simulink model "qubeLQGR_discrete_distrej"  (R2024b)
settings: Solver=ode1  StartTime=0.0  StopTime=120  RelTol=1e-3  EnableMultiTasking=on
values from neighbouring files (symbols this model uses):
  epsilon = 0.00242    [MPC_controller.m]    (also in MPC_controller_withint_testing.m)
  h = log(abs(sec(theta)+tan(theta))-C1*alpha)    [Design_of_nonlinear_controller.m]    (also in MPC_controller.m = 0.01; MPC_controller_withint_testing.m = 0.01)
undefined symbols (not defined in the file or in its folder): Discrete, Humusoft, MF634, Time
libraries: sldrtlib x2, simulink x2, ctrlSharedLib x1
settings Model: Creator=rbabuska  LastModifiedBy=Wesley
settings SolverCC: AlgebraicLoopSolver=TrustRegion
settings DataIOCC: LimitDataPoints=on  SaveFormat=Array  SignalLoggingSaveFormat=ModelDataLogs  ReturnWorkspaceOutputs=off
settings OptimizationCC: ExpressionDepthLimit=2147483647  LifeSpan=inf
settings DebuggingCC: UnderspecifiedInitializationDetection=Classic  MergeDetectMultiDrivingBlocksExec=none  FcnCallInpInsideContextMsg=warning  UnconnectedInputMsg=warning  UnconnectedOutputMsg=warning  UnconnectedLineMsg=warning  StateNameClashWarn=warning  SFUnexpectedBacktrackingDiag=warning  SFNoUnconditionalDefaultTransitionDiag=warning  SFExecutionAtInitializationDiag=none  ArithmeticOperatorsInVariantConditions=warning
settings HardwareCC: ProdBitPerPointer=32  ProdBitPerSizeT=32  ProdBitPerPtrDiffT=32  ProdLargestAtomicFloat=None  ProdIntDivRoundTo=Undefined  ProdEndianess=Unspecified  ProdWordSize=32  ProdHWDeviceType=32-bit Generic
settings ModelReferenceCC: EnableRefExpFcnMdlSchedulingChecks=on  PropagateSignalLabelsOutOfModel=off
settings SFSimCC: SimUseLocalCustomCode=off  CustomCodeUndefinedFunction=UseInterfaceOnly
settings RTWCC: RTWUseLocalCustomCode=off  GPUComputeCapability=3.5  DLArmComputeVersion=19.05
settings CodeAppCC: StateflowObjectComments=on
settings GRTTargetCC: TargetLangStandard=C89/C90 (ANSI)  CombineOutputUpdateFcns=off  GRTInterface=on
settings ConfigComp: CovMetricSettings=dw  CovSaveCumulativeToWorkspaceVar=on  CovSaveSingleToWorkspaceVar=on  CovExternalEMLEnable=off  CovSFcnEnable=off

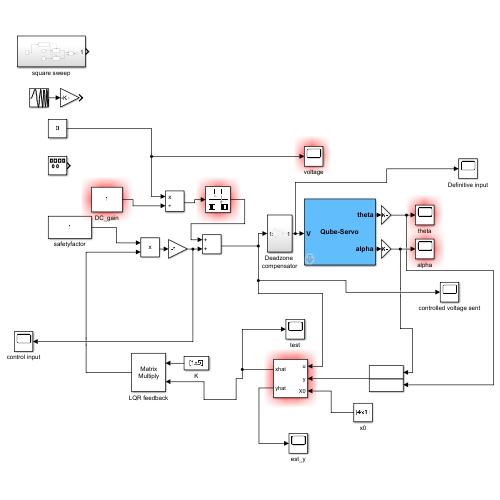
[thumbnail: Simulink's stored preview of the top-level diagram]
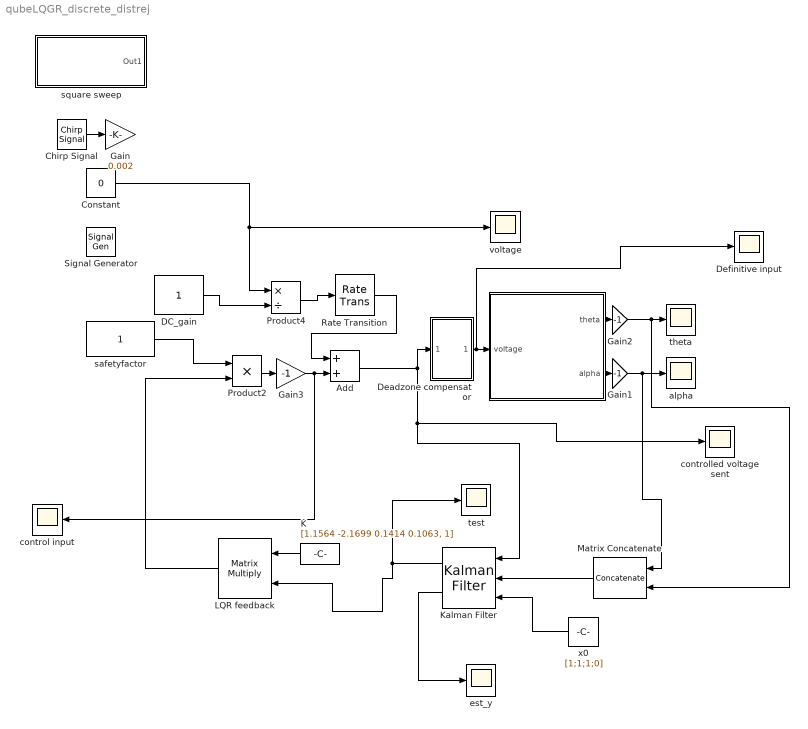
== system qubeLQGR_discrete_distrej ==
  " " : Subsystem  LoadFcn=hwinit  InitFcn=hwinit  mask{h=h}
      mask prompts: h "Sampling period [s]"
      mask Display:
      | disp('Qube-Servo')
      | port_label('output',1,'theta')
      | port_label('output',2,'alpha')
      | port_label('input',1,'V')
  Add : Sum  RndMeth=Nearest
  Chirp Signal : simulink/Sources/Chirp Signal  f1=0  T=120  f2=5
  Constant : Constant  Value=0
  DC_gain : Constant  SampleTime=h
  Deadzone compensator : Subsystem
  Definitive input : Scope
  Gain : Gain  Gain=0.002
  Gain1 : Gain  Gain=-1
  Gain2 : Gain  Gain=-1
  Gain3 : Gain  Gain=-1
  K : Constant  Value=[1.1564 -2.1699 0.1414 0.1063, 1]  VectorParams1D=off
  Kalman Filter : ctrlSharedLib/Kalman Filter  TimeDomain=Discrete-Time  UseCurrentEstimator=on  ModelSource=Individual A, B, C, D matrices  ModelSourceVariable=ss(0.95,1,1,0,1)  A=[0.9989,0.005226,0.009805,0.00007506,0;0.001157,0.9886,0.00004467,0.009909,0;-0.2158,1.032,0.961,0.01663,0;0.2302,-2.268,0.009227,0.978,0;0,0,0,0,1]  B=[0.1529;-0.145;30.29;-28.85;0]  C=[1,0,0,0,0;0,1,0,0,0]  D=[0;0]  NumberOfStates=1  NumberOfInputs=1  NumberOfOutputs=1  InitialEstimateSource=Input port  X0=0  P0=10  UseK=off  UseGH=off  NumberOfProcessNoiseInputs=1  G=1  TimeInvariantG=on  H=0  TimeInvariantH=on  Q=blkdiag(6*(1e-5)*eye(4), 1e-2)  TimeInvariantQ=on  R=1e-10  TimeInvariantR=on  N=0  TimeInvariantN=on  AddInputPort=on  AddEnablePort=off  OutputEstimatedY=on  OutputP=off  Ts=h
  LQR feedback : Product  Multiplication=Matrix(*)
  Matrix Concatenate : Concatenate  ConcatenateDimension=2
  Product2 : Product
  Product4 : Product  Inputs=*/
  Rate Transition : RateTransition  OutPortSampleTime=h
  Signal Generator : SignalGenerator  WaveForm=square  Amplitude=0  Frequency=0.1
  alpha : Scope
  control input : Scope
  controlled voltage sent : Scope
  est_y : Scope
  safetyfactor : Constant
  square sweep : Subsystem
  test : Scope
  theta : Scope
  voltage : Scope
  x0 : Constant  Value=[1;1;1;0]
  wires:
  Gain2/1 -> Matrix Concatenate/2, theta/1
  Matrix Concatenate/1 -> Kalman Filter/2
  K/1 -> LQR feedback/1
  Kalman Filter/1 -> LQR feedback/2, test/1
  safetyfactor/1 -> Product2/1
  Kalman Filter/2 -> est_y/1
  LQR feedback/1 -> Product2/2
  DC_gain/1 -> Product4/2
  Product4/1 -> Rate Transition/1
  Deadzone compensator/1(Out1) -> Definitive input/1, " "/1(voltage)
  Gain1/1 -> Matrix Concatenate/1, alpha/1
  Constant/1 -> Product4/1, voltage/1
  " "/2(alpha) -> Gain1/1
  " "/1(theta) -> Gain2/1
  Chirp Signal/1 -> Gain/1
  x0/1 -> Kalman Filter/3
  Product2/1 -> Gain3/1
  Gain3/1 -> control input/1, Add/2
  Rate Transition/1 -> Add/1
  Add/1 -> controlled voltage sent/1, Kalman Filter/1, Deadzone compensator/1(In1)

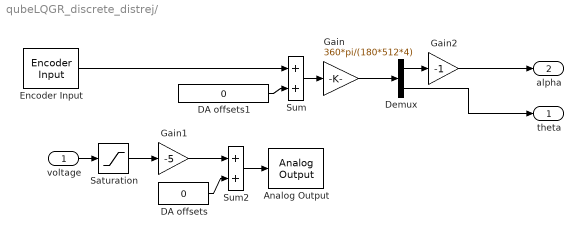
== system qubeLQGR_discrete_distrej/  ==
  voltage : Inport
  Analog Output : sldrtlib/Analog Output  SampleTime=h  MaxMissedTicks=100  ShowMissedTicks=off  YieldWhenWaiting=off  DrvName=Humusoft/MF634  DrvAddress=4294967295  DrvOptions=0  Channels=[1]  RangeMode=2  VoltRange=1  InitialValue=0  FinalValue=0
      settings: AttributesFormatString=Humusoft\nMF634 [auto]
  DA offsets : Constant  Value=0
  DA offsets1 : Constant  Value=0  SampleTime=h
  Demux : Demux  Outputs=2
  Encoder Input : sldrtlib/Encoder Input  SampleTime=h  MaxMissedTicks=100  ShowMissedTicks=off  YieldWhenWaiting=off  DrvName=Humusoft/MF634  DrvAddress=4294967295  DrvOptions=0  Channels=[1,2]  QuadMode=3  IndexPulse=1  InputFilter=Inf  DataType=1
      settings: AttributesFormatString=Humusoft\nMF634 [auto]
  Gain : Gain  Gain=360*pi/(180*512*4)  SaturateOnIntegerOverflow=on  OutDataTypeStr=Inherit: Same as input  ParamDataTypeStr=Inherit: Same as input
  Gain1 : Gain  Gain=-5  SaturateOnIntegerOverflow=on  OutDataTypeStr=Inherit: Same as input  ParamDataTypeStr=Inherit: Same as input
  Gain2 : Gain  Gain=-1  SaturateOnIntegerOverflow=on  OutDataTypeStr=Inherit: Same as input  ParamDataTypeStr=Inherit: Same as input
  Saturation : Saturate  UpperLimit=1  LowerLimit=-1
  Sum : Sum  InputSameDT=on  SaturateOnIntegerOverflow=on  OutDataTypeStr=Inherit: Same as first input
  Sum2 : Sum  InputSameDT=on  SaturateOnIntegerOverflow=on  OutDataTypeStr=Inherit: Same as first input
  theta : Outport  Tag=Cable length
  alpha : Outport  Tag=Cable length  Port=2
  wires:
  Sum/1 -> Gain/1
  DA offsets1/1 -> Sum/2
  Gain1/1 -> Sum2/1
  Sum2/1 -> Analog Output/1
  DA offsets/1 -> Sum2/2
  voltage/1 -> Saturation/1
  Encoder Input/1 -> Sum/1
  Saturation/1 -> Gain1/1
  Demux/1 -> Gain2/1
  Gain/1 -> Demux/1
  Gain2/1 -> alpha/1
  Demux/2 -> theta/1

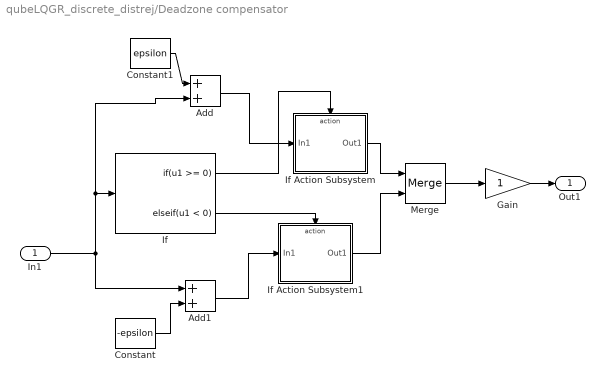
== system qubeLQGR_discrete_distrej/Deadzone compensator ==
  In1 : Inport
  Add : Sum
  Add1 : Sum
  Constant : Constant  Value=-epsilon
  Constant1 : Constant  Value=epsilon
  Gain : Gain
  If : If  IfExpression=u1 >= 0  ElseIfExpressions=u1 < 0  ShowElse=off
  If Action Subsystem : Subsystem  TreatAsAtomicUnit=on
  If Action Subsystem1 : Subsystem  TreatAsAtomicUnit=on
  Merge : Merge
  Out1 : Outport
  wires:
  If Action Subsystem/1(Out1) -> Merge/1
  Gain/1 -> Out1/1
  Merge/1 -> Gain/1
  If/2 -> If Action Subsystem1/Action
  Add/1 -> If Action Subsystem/1(In1)
  If/1 -> If Action Subsystem/Action
  If Action Subsystem1/1(Out1) -> Merge/2
  In1/1 -> Add1/1, Add/2, If/1
  Constant1/1 -> Add/1
  Constant/1 -> Add1/2
  Add1/1 -> If Action Subsystem1/1(In1)

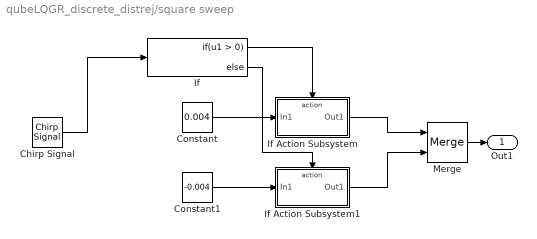
== system qubeLQGR_discrete_distrej/square sweep ==
  Chirp Signal : simulink/Sources/Chirp Signal  f1=0  T=120  f2=5
  Constant : Constant  Value=0.004
  Constant1 : Constant  Value=-0.004
  If : If
  If Action Subsystem : Subsystem  TreatAsAtomicUnit=on
  If Action Subsystem1 : Subsystem  TreatAsAtomicUnit=on
  Merge : Merge
  Out1 : Outport
  wires:
  Merge/1 -> Out1/1
  If/2 -> If Action Subsystem1/Action
  Chirp Signal/1 -> If/1
  Constant/1 -> If Action Subsystem/1(In1)
  If Action Subsystem1/1(Out1) -> Merge/2
  If Action Subsystem/1(Out1) -> Merge/1
  If/1 -> If Action Subsystem/Action
  Constant1/1 -> If Action Subsystem1/1(In1)

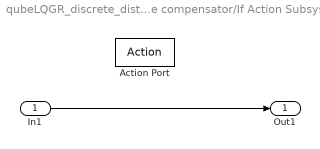
== system qubeLQGR_discrete_distrej/Deadzone compensator/If Action Subsystem ==
  In1 : Inport
  Action Port : ActionPort  ActionPortLabel=if(u1 >= 0)
  Out1 : Outport
  wires:
  In1/1 -> Out1/1

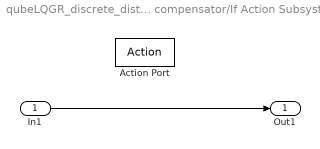
== system qubeLQGR_discrete_distrej/Deadzone compensator/If Action Subsystem1 ==
  In1 : Inport
  Action Port : ActionPort  ActionPortLabel=elseif(u1 < 0)
  Out1 : Outport
  wires:
  In1/1 -> Out1/1

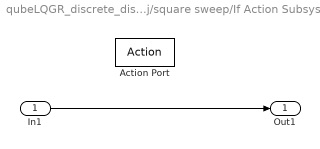
== system qubeLQGR_discrete_distrej/square sweep/If Action Subsystem ==
  In1 : Inport
  Action Port : ActionPort  ActionPortLabel=if(u1 > 0)
  Out1 : Outport
  wires:
  In1/1 -> Out1/1

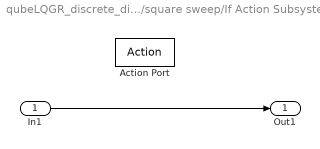
== system qubeLQGR_discrete_distrej/square sweep/If Action Subsystem1 ==
  In1 : Inport
  Action Port : ActionPort  ActionPortLabel=else
  Out1 : Outport
  wires:
  In1/1 -> Out1/1
